simulink library "invLib"  (R2026a)
settings: Solver=VariableStepAuto
values from neighbouring files (symbols this model uses):
  ip = invParams()    [invSim.m]    (also in inv_current_loop_check.m; inv_grid_thd_check.m; inv_model_check.m; inv_thd_check.m)
libraries: nesl_utility x15, ee_lib x9, fl_lib x9, slpidlib x2
settings Model: Creator=phamn  LastModifiedBy=phamn

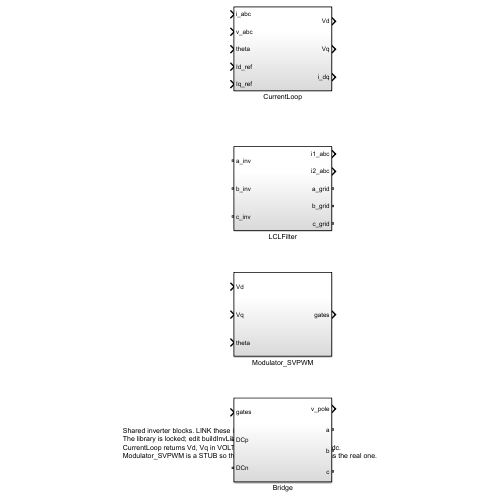
[thumbnail: Simulink's stored preview of the top-level diagram]
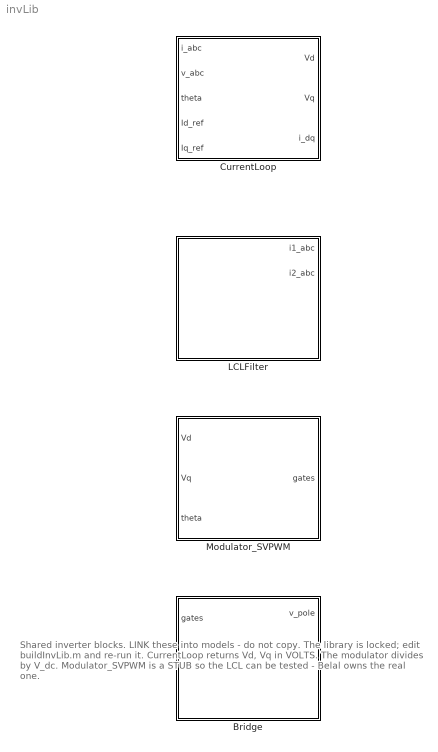
== system invLib ==
  note: Shared inverter blocks. LINK these into models - do not copy.
      | The library is locked; edit buildInvLib.m and re-run it.
      | CurrentLoop returns Vd, Vq in VOLTS. The modulator divides by V_dc.
      | Modulator_SVPWM is a STUB so the LCL can be tested - Belal owns the real one.
  Bridge : Subsystem
  CurrentLoop : Subsystem
  LCLFilter : Subsystem
  Modulator_SVPWM : Subsystem

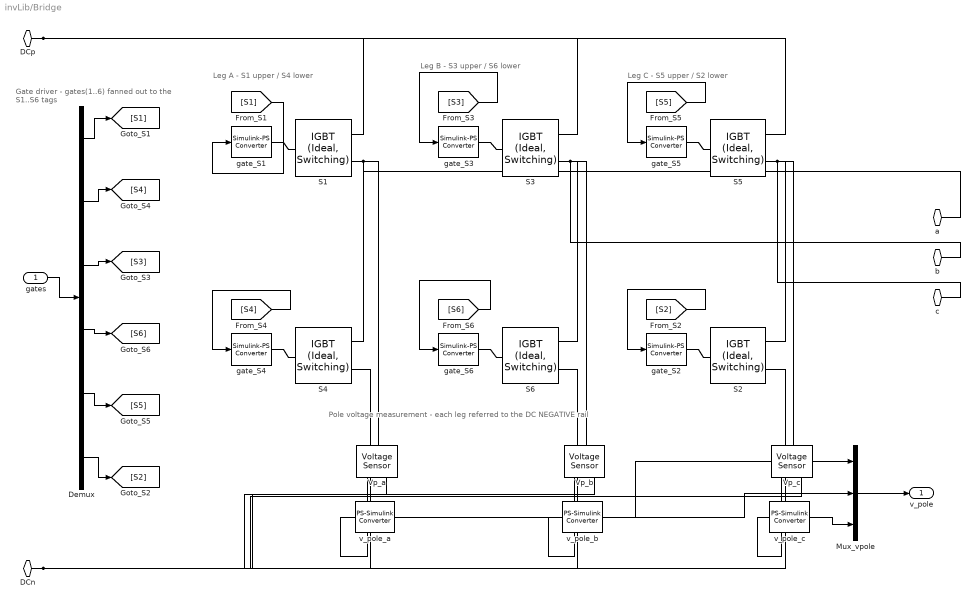
== system invLib/Bridge ==
  note: Gate driver - gates(1..6) fanned out to the S1..S6 tags
  note: Leg A - S1 upper / S4 lower
  note: Leg B - S3 upper / S6 lower
  note: Leg C - S5 upper / S2 lower
  note: Pole voltage measurement - each leg referred to the DC NEGATIVE rail
  gates : Inport
  Demux : Demux  Outputs=6
  Mux_vpole : Mux  Inputs=3
  S{1..6} (6 alike) : ee_lib/Semiconductors & Converters/IGBT (Ideal, Switching)  port_option=ee.enum.controlport.ps  Vf=ip.Vf_dev V  Ron=ip.Ron_dev Ohm  Goff=ip.Goff_dev 1/Ohm  Vth=ip.Vth_gate V  diode_param=ee.enum.semiconductors.protectionDiode.nodynamics  diode_Vf=ip.Vf_dev V  diode_Ron=ip.Ron_dev Ohm  diode_Goff=ip.Goff_dev 1/Ohm  diode_C=50e-9 F  diode_iRM=-235 A  diode_iF=300 A  diode_idot=-50 A/us  diode_trr_param=ee.enum.converters.diodeReverseParam.trr_factor  diode_trr_factor=3  diode_trr=15 us  diode_Qrr=1500 s*uA  ice_specify=off  ice_priority=None  ice=0 A  ice_nominal_specify=off  ice_nominal_value=1  ice_nominal_unit=A  vce_specify=off  vce_priority=None  vce=0 V  vce_nominal_specify=off  vce_nominal_value=1  vce_nominal_unit=V  vge_specify=off  vge_priority=None  vge=0 V  vge_nominal_specify=off  vge_nominal_value=1  vge_nominal_unit=V  thermal_loss_option=ee.enum.converters.thermalLossOption.constantvalues  Von_data=[0, .1, .6, .8, 1, 1.3, 1.6, 2, 2.4; 0, .1, .7, 1, 1.2, 1.5, 1.9, 2.4, 2.8] V  Tj=[298.15, 398.15] K  Iout_data=[0, .1, 1, 5, 10, 20, 40, 70, 100] A  tabulateWithVce=false  Eon_data=[0, .0024, .024, .12, .2, .48, 1.04, 2.16, 3.24; 0, .003, .03, .15, .25, .6, 1.3, 2.7, 4.05] * 1e-3 J  Eoff_data=[0, .0007, .0066, .033, .066, .17, .33, .83, 1.5; 0, .001, .01, .05, .1, .25, .5, 1.2, 2.2] * 1e-3 J  Eon_data_3D=[zeros(2, 9, 3)] J  Eoff_data_3D=[zeros(2, 9, 3)] J  Tj_loss=[298.15, 398.15] K  Iout_data_loss=[0, .1, 1, 5, 10, 20, 40, 70, 100] A  Vce_loss=[0, 150, 300] V  Eon_scalar=22.86e-3 J  Eoff_scalar=17.14e-3 J  Voff=300 V  Iout_scalar=600 A  useCurrentFromPreviousCycle=false  useVoltageFromPreviousCycle=false  diodeModelType=ee.enum.converters.diodeModelType.pwl  diodeTableType=ee.enum.diode.tableType.IfMat  diode_ReverseIVType=ee.enum.diode.diodeReverseIV.constant  diode_IfMat=[.07, .12, .19, 1.75, 4.24, 7.32, 11.2; .16, .3, .72, 2.14, 4.02, 6.35, 9.12] A  diode_VfMat=[.9, 1.15, 1.25, 1.5, 1.75, 2.17, 2.6, 2.85; .58, .68, .75, 1.1, 1.38, 1.77, 2.27, 2.7] V  diode_TjVec=[25, 125] degC  diode_VfVec=[.5, .7, .9, 1.3, 1.7, 2.1, 2.5] V  diode_IfVec=[.1, .2, .5, 1, 2, 4, 7, 10] A  diode_IrMat=[1e-06, 2e-06, 5e-06, 1e-05, 2.5e-05, 5e-05, .0001; 2e-06, 5e-06, 1e-05, 4e-05, 8e-05, .0002, .0005] A  diode_VrMat=[10, 100, 200, 250, 300, 325, 350; 10, 70, 160, 220, 270, 300, 320] V  diode_VrVec=[10, 20, 40, 50, 70, 80, 100] V  diode_IrVec=[1e-06, 2e-06, 5e-06, 1e-05, 2e-05, 5e-05, .0001] A  diode_Vr=-600 V  diode_Ls=150 nH  diode_Erec=0.03 J  diode_rec_loss_model=ee.enum.diode.reverseRecoveryModelTabulateUpTo3D.fixed  diode_ErecVal=0 J  diode_scaleWithIandV=true  diode_ErecMat=zeros(2, 3) J  diodeErecMat3D=zeros(2, 3, 2) J  diode_TjrecVec=[298.15, 398.15] K  diode_IfrecVec=[.1, 1, 10] A  diodeVrecVec=[0, 100] V  diode_IrecVal=10 A  diode_VrecVal=10 V  diode_tFilter=1 / 1000 / 100 s  separateThermalPortForDiode=false  thermal_network_parameterization=ee.enum.thermalNetworkTopology.external  Rth=[.08, .5] K/W  Rth_Cauer=[.08, .1, .5] K/W  Rth_Foster=[.08, .14, .22, .16] K/W  thermal_mass_parameterization=ee.enum.thermalNetwork.timeconstant  thermal_mass=[.01, .5] J/K  thermal_mass_Cauer=[.01, .1, .5] J/K  thermal_mass_Foster=[.001, .005, .05, .5] J/K  thermal_time_constant=[.001, .2] s  thermal_time_constant_Cauer=[.001, .1, .2] s  thermal_time_constant_Foster=[7e-05, .0007, .01, .08] s  thermal_mass_initial_temperatures=[25, 25] degC  thermal_mass_initial_temperatures_Cauer=[25, 25, 25] degC  junction_thermal_mass=0.01 J/K  Tvec_initial_Foster=[25, 25, 25, 25] degC  RthDiode=[.03, .2] K/W  RthCauerDiode=[.03, .1, .2] K/W  RthFosterDiode=[.03, .2] K/W  thermalMassDiode=[3, 25] J/K  thermalMassCauerDiode=[3, 10, 25] J/K  thermalMassFosterDiode=[33, 50] J/K  thermalTauDiode=[.1, 5] s  thermalTauCauerDiode=[.1, 1, 5] s  thermalTauFosterDiode=[1, 10] s  thermalMassInitTempDiode=[25, 25] degC  thermalMassInitTempCauerDiode=[25, 25, 25] degC  junctionthermalMassDiode=0.1 J/K  TVecInitialFosterDiode=[25, 25, 25, 25] degC  no_thermal_network=ee.enum.enable.no  IGBT_junction_temperature_specify=off  IGBT_junction_temperature_priority=None  IGBT_junction_temperature=25 degC  IGBT_junction_temperature_nominal_specify=off  IGBT_junction_temperature_nominal_value=1  IGBT_junction_temperature_nominal_unit=degC  diode_junction_temperature_specify=off  diode_junction_temperature_priority=None  diode_junction_temperature=25 degC  diode_junction_temperature_nominal_specify=off  diode_junction_temperature_nominal_value=1  diode_junction_temperature_nominal_unit=degC  Qj_specify=off  Qj_priority=None  Qj=0 W  Qj_nominal_specify=off  Qj_nominal_value=1  Qj_nominal_unit=W  accumulatedSwitchingLosses_specify=off  accumulatedSwitchingLosses_priority=None  accumulatedSwitchingLosses=0 J
  Vp_a : fl_lib/Electrical/Electrical Sensors/Voltage Sensor
  Vp_b : fl_lib/Electrical/Electrical Sensors/Voltage Sensor
  Vp_c : fl_lib/Electrical/Electrical Sensors/Voltage Sensor
  gate_S{1..6} (6 alike) : nesl_utility/Simulink-PS Converter  PhysicalDomain=network_engine_domain  SubClassName=ps_input  LeftPortType=input  RightPortType=output  PseudoPeriodic=off  Frequencies=[]  NoiseDistribution=none  NoiseParameters=[]  Unit=1  AffineConversion=off  FilteringAndDerivatives=provide  SimscapeFilterOrder=1  InputFilterTimeConstant=0.001  UdotUserProvided=0
  v_pole_a : nesl_utility/PS-Simulink Converter  PhysicalDomain=network_engine_domain  SubClassName=ps_output  LeftPortType=input  RightPortType=output  PseudoPeriodic=off  Frequencies=[]  VectorFormat=inherit  Unit=inherit  AffineConversion=off
  v_pole_b : nesl_utility/PS-Simulink Converter  PhysicalDomain=network_engine_domain  SubClassName=ps_output  LeftPortType=input  RightPortType=output  PseudoPeriodic=off  Frequencies=[]  VectorFormat=inherit  Unit=inherit  AffineConversion=off
  v_pole_c : nesl_utility/PS-Simulink Converter  PhysicalDomain=network_engine_domain  SubClassName=ps_output  LeftPortType=input  RightPortType=output  PseudoPeriodic=off  Frequencies=[]  VectorFormat=inherit  Unit=inherit  AffineConversion=off
  DCp : PMIOPort  Side=Left
  DCn : PMIOPort  Port=2  Side=Left
  a : PMIOPort  Port=3  Side=Right
  b : PMIOPort  Port=4  Side=Right
  c : PMIOPort  Port=5  Side=Right
  v_pole : Outport
  wires:
  gates/1 -> Demux/1
  Demux/1 -> [S1]
  Demux/2 -> [S4]
  Demux/3 -> [S3]
  Demux/4 -> [S6]
  Demux/5 -> [S5]
  Demux/6 -> [S2]
  [S1] -> gate_S1/1
  [S4] -> gate_S4/1
  v_pole_a/1 -> Mux_vpole/1
  [S3] -> gate_S3/1
  [S6] -> gate_S6/1
  v_pole_b/1 -> Mux_vpole/2
  [S5] -> gate_S5/1
  [S2] -> gate_S2/1
  v_pole_c/1 -> Mux_vpole/3
  Mux_vpole/1 -> v_pole/1
  connections:
  gate_S1/RConn1 -- S1/LConn1
  gate_S4/RConn1 -- S4/LConn1
  S1/RConn1 -- DCp/RConn1 -- S3/RConn1 -- S5/RConn1
  S4/RConn1 -- S1/RConn2 -- a/RConn1 -- Vp_a/LConn1
  S4/RConn2 -- Vp_a/RConn2 -- S6/RConn2 -- Vp_b/RConn2 -- S2/RConn2 -- DCn/RConn1 -- Vp_c/RConn2
  Vp_a/RConn1 -- v_pole_a/LConn1
  gate_S3/RConn1 -- S3/LConn1
  gate_S6/RConn1 -- S6/LConn1
  S6/RConn1 -- S3/RConn2 -- b/RConn1 -- Vp_b/LConn1
  Vp_b/RConn1 -- v_pole_b/LConn1
  gate_S5/RConn1 -- S5/LConn1
  gate_S2/RConn1 -- S2/LConn1
  S2/RConn1 -- S5/RConn2 -- c/RConn1 -- Vp_c/LConn1
  Vp_c/RConn1 -- v_pole_c/LConn1

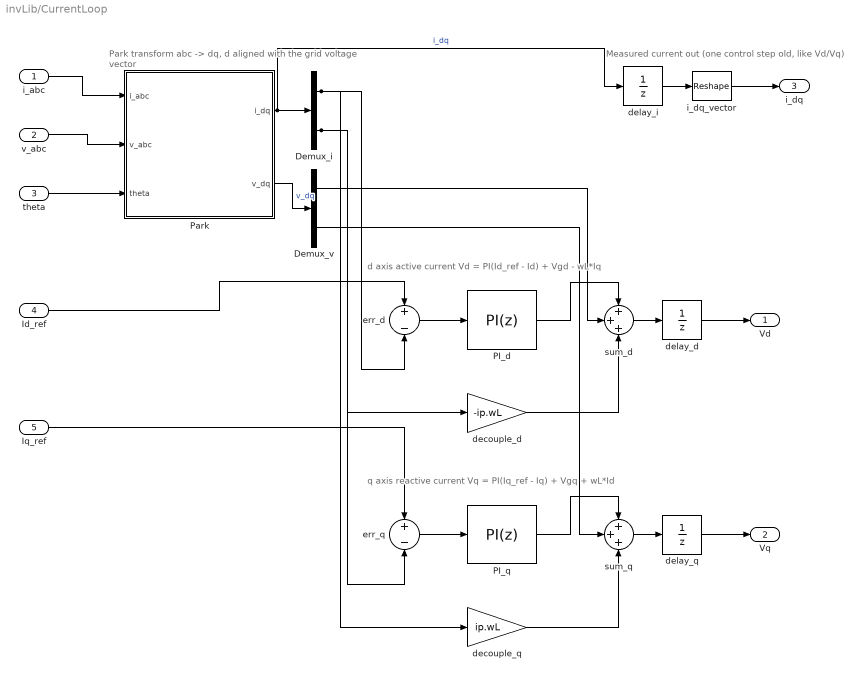
== system invLib/CurrentLoop ==
  note: Park transform abc -> dq, d aligned with the grid voltage vector
  note: d axis active current Vd = PI(Id_ref - Id) + Vgd - wL*Iq
  note: q axis reactive current Vq = PI(Iq_ref - Iq) + Vgq + wL*Id
  note: Measured current out (one control step old, like Vd/Vq)
  i_abc : Inport
  v_abc : Inport  Port=2
  theta : Inport  Port=3
  Id_ref : Inport  Port=4
  Iq_ref : Inport  Port=5
  Demux_i : Demux  Outputs=2
  Demux_v : Demux  Outputs=2
  PI_d : slpidlib/PID Controller  Controller=PI  Form=Parallel  TimeDomain=Discrete-time  UseExternalTs=off  SampleTime=ip.Ts_ctrl  IntegratorMethod=Backward Euler  FilterMethod=Forward Euler  ControllerParametersSource=internal  P=ip.Kp_i  I=ip.Ki_i  UseKiTs=off  D=0  UseExternalDerivativeSource=off  N=100  UseFilter=on  TunerSelectOption=Transfer Function Based (PID Tuner App)  InitialConditionSource=internal  InitialConditionForIntegrator=0  InitialConditionForFilter=0  DifferentiatorICPrevScaledInput=0  ExternalReset=none  TrackingMode=off  Kt=1  LimitOutput=on  SatLimitsSource=internal  UpperSaturationLimit=ip.V_pi_max  LowerSaturationLimit=-ip.V_pi_max  LinearizeAsGain=off  AntiWindupMode=clamping  Kb=1  LimitIntegrator=off  UpperIntegratorSaturationLimit=inf  LowerIntegratorSaturationLimit=-inf  POutMin=[]  POutMax=[]  IOutMin=[]  IOutMax=[]  DOutMin=[]  DOutMax=[]  NOutMin=[]  NOutMax=[]  SumOutMin=[]  SumOutMax=[]  SaturationOutMin=[]  SaturationOutMax=[]  PParamMin=[]  PParamMax=[]  IParamMin=[]  IParamMax=[]  DParamMin=[]  DParamMax=[]  NParamMin=[]  NParamMax=[]  KbParamMin=[]  KbParamMax=[]  KtParamMin=[]  KtParamMax=[]  KbOutMin=[]  KbOutMax=[]  KtOutMin=[]  KtOutMax=[]  IntegratorOutMin=[]  IntegratorOutMax=[]  FilterOutMin=[]  FilterOutMax=[]  SumI1OutMin=[]  SumI1OutMax=[]  SumI2OutMin=[]  SumI2OutMax=[]  SumI3OutMin=[]  SumI3OutMax=[]  SumI4OutMin=[]  SumI4OutMax=[]  SumDOutMin=[]  SumDOutMax=[]  DifferentiatorOutMin=[]  DifferentiatorOutMax=[]  FilterDiffOutCoefMin=[]  FilterDiffOutCoefMax=[]  ReciprocalOutMin=[]  ReciprocalOutMax=[]  SumDenOutMin=[]  SumDenOutMax=[]  SumNumOutMin=[]  SumNumOutMax=[]  DivideOutMin=[]  DivideOutMax=[]  UdiffTsProdOutMin=[]  UdiffTsProdOutMax=[]  NTsProdOutMin=[]  NTsProdOutMax=[]  UintegralTsProdOutMin=[]  UintegralTsProdOutMax=[]  UngainTsProdOutMin=[]  UngainTsProdOutMax=[]  ClampingZeroOutDataTypeStr=Inherit: Inherit via back propagation  ClampingZeroOutMin=[]  ClampingZeroOutMax=[]  FilterDenConstantOutDataTypeStr=Inherit: Inherit via back propagation  FilterDenConstantOutMin=[]  FilterDenConstantOutMax=[]  PCopyOutDataTypeStr=Inherit: Inherit via back propagation  PCopyOutMin=[]  PCopyOutMax=[]  NCopyOutDataTypeStr=Inherit: Inherit via back propagation  NCopyOutMin=[]  NCopyOutMax=[]  IntegratorContinuousStateAttributes=''  IntegratorStateMustResolveToSignalObject=off  IntegratorRTWStateStorageClass=Auto  FilterContinuousStateAttributes=''  FilterStateMustResolveToSignalObject=off  FilterRTWStateStorageClass=Auto  ParallelPVariant=InternalParameters  IdealPVariant=Disabled  IVariant=InternalParameters  DVariant=Disabled  IntegratorVariant=Discrete  SatVariant=Enabled  AWVariant=DiscClampingParallel  PCopyVariant=Disabled  TRVariant=Disabled  FdbkBlocksVariant=Feedback  IdealPFdbkVariant=Passthrough  SatFdbkVariant=Passthrough  DerivativeFilterVariant=Disabled  NVariant=Disabled  NCopyVariant=Disabled_SignalSpec  FilterICVariant=Disabled  IntegratorICVariant=InternalICs  ExternalResetVariant=Disabled  TRSumVariant=Passthrough  SumFdbkVariant=Enabled  SumVariant=Sum_PI  TsampFilterVariant=InternalTs  TsampNgainVariant=Passthrough  TsampIntegralVariant=Disabled_SignalSpec  ExternalSaturationOutDataTypeStr=Inherit: Same as second input  DerivativeSourceVariant=Disabled  PreIntVariant=InternalPreInt
      settings: LibrarySourceBlock=simulink/Discrete/Discrete PID Controller
  PI_q : slpidlib/PID Controller  Controller=PI  Form=Parallel  TimeDomain=Discrete-time  UseExternalTs=off  SampleTime=ip.Ts_ctrl  IntegratorMethod=Backward Euler  FilterMethod=Forward Euler  ControllerParametersSource=internal  P=ip.Kp_i  I=ip.Ki_i  UseKiTs=off  D=0  UseExternalDerivativeSource=off  N=100  UseFilter=on  TunerSelectOption=Transfer Function Based (PID Tuner App)  InitialConditionSource=internal  InitialConditionForIntegrator=0  InitialConditionForFilter=0  DifferentiatorICPrevScaledInput=0  ExternalReset=none  TrackingMode=off  Kt=1  LimitOutput=on  SatLimitsSource=internal  UpperSaturationLimit=ip.V_pi_max  LowerSaturationLimit=-ip.V_pi_max  LinearizeAsGain=off  AntiWindupMode=clamping  Kb=1  LimitIntegrator=off  UpperIntegratorSaturationLimit=inf  LowerIntegratorSaturationLimit=-inf  POutMin=[]  POutMax=[]  IOutMin=[]  IOutMax=[]  DOutMin=[]  DOutMax=[]  NOutMin=[]  NOutMax=[]  SumOutMin=[]  SumOutMax=[]  SaturationOutMin=[]  SaturationOutMax=[]  PParamMin=[]  PParamMax=[]  IParamMin=[]  IParamMax=[]  DParamMin=[]  DParamMax=[]  NParamMin=[]  NParamMax=[]  KbParamMin=[]  KbParamMax=[]  KtParamMin=[]  KtParamMax=[]  KbOutMin=[]  KbOutMax=[]  KtOutMin=[]  KtOutMax=[]  IntegratorOutMin=[]  IntegratorOutMax=[]  FilterOutMin=[]  FilterOutMax=[]  SumI1OutMin=[]  SumI1OutMax=[]  SumI2OutMin=[]  SumI2OutMax=[]  SumI3OutMin=[]  SumI3OutMax=[]  SumI4OutMin=[]  SumI4OutMax=[]  SumDOutMin=[]  SumDOutMax=[]  DifferentiatorOutMin=[]  DifferentiatorOutMax=[]  FilterDiffOutCoefMin=[]  FilterDiffOutCoefMax=[]  ReciprocalOutMin=[]  ReciprocalOutMax=[]  SumDenOutMin=[]  SumDenOutMax=[]  SumNumOutMin=[]  SumNumOutMax=[]  DivideOutMin=[]  DivideOutMax=[]  UdiffTsProdOutMin=[]  UdiffTsProdOutMax=[]  NTsProdOutMin=[]  NTsProdOutMax=[]  UintegralTsProdOutMin=[]  UintegralTsProdOutMax=[]  UngainTsProdOutMin=[]  UngainTsProdOutMax=[]  ClampingZeroOutDataTypeStr=Inherit: Inherit via back propagation  ClampingZeroOutMin=[]  ClampingZeroOutMax=[]  FilterDenConstantOutDataTypeStr=Inherit: Inherit via back propagation  FilterDenConstantOutMin=[]  FilterDenConstantOutMax=[]  PCopyOutDataTypeStr=Inherit: Inherit via back propagation  PCopyOutMin=[]  PCopyOutMax=[]  NCopyOutDataTypeStr=Inherit: Inherit via back propagation  NCopyOutMin=[]  NCopyOutMax=[]  IntegratorContinuousStateAttributes=''  IntegratorStateMustResolveToSignalObject=off  IntegratorRTWStateStorageClass=Auto  FilterContinuousStateAttributes=''  FilterStateMustResolveToSignalObject=off  FilterRTWStateStorageClass=Auto  ParallelPVariant=InternalParameters  IdealPVariant=Disabled  IVariant=InternalParameters  DVariant=Disabled  IntegratorVariant=Discrete  SatVariant=Enabled  AWVariant=DiscClampingParallel  PCopyVariant=Disabled  TRVariant=Disabled  FdbkBlocksVariant=Feedback  IdealPFdbkVariant=Passthrough  SatFdbkVariant=Passthrough  DerivativeFilterVariant=Disabled  NVariant=Disabled  NCopyVariant=Disabled_SignalSpec  FilterICVariant=Disabled  IntegratorICVariant=InternalICs  ExternalResetVariant=Disabled  TRSumVariant=Passthrough  SumFdbkVariant=Enabled  SumVariant=Sum_PI  TsampFilterVariant=InternalTs  TsampNgainVariant=Passthrough  TsampIntegralVariant=Disabled_SignalSpec  ExternalSaturationOutDataTypeStr=Inherit: Same as second input  DerivativeSourceVariant=Disabled  PreIntVariant=InternalPreInt
      settings: LibrarySourceBlock=simulink/Discrete/Discrete PID Controller
  Park : MATLAB Function  TreatAsAtomicUnit=on
  decouple_d : Gain  Gain=-ip.wL
  decouple_q : Gain  Gain=ip.wL
  delay_d : UnitDelay  SampleTime=ip.Ts_ctrl
  delay_i : UnitDelay  SampleTime=ip.Ts_ctrl
  delay_q : UnitDelay  SampleTime=ip.Ts_ctrl
  err_d : Sum  Inputs=+-
  err_q : Sum  Inputs=+-
  i_dq_vector : Reshape
  sum_d : Sum  Inputs=+++
  sum_q : Sum  Inputs=+++
  Vd : Outport
  Vq : Outport  Port=2
  i_dq : Outport  Port=3
  wires:
  i_abc/1 -> Park/1(i_abc)
  v_abc/1 -> Park/2(v_abc)
  theta/1 -> Park/3(theta)
  Park/1(i_dq) -> Demux_i/1, delay_i/1  "i_dq"
  Park/2(v_dq) -> Demux_v/1  "v_dq"
  Id_ref/1 -> err_d/1
  Demux_i/1 -> err_d/2, decouple_q/1
  Iq_ref/1 -> err_q/1
  Demux_i/2 -> err_q/2, decouple_d/1
  err_d/1 -> PI_d/1
  err_q/1 -> PI_q/1
  PI_d/1 -> sum_d/1
  Demux_v/1 -> sum_d/2
  decouple_d/1 -> sum_d/3
  PI_q/1 -> sum_q/1
  Demux_v/2 -> sum_q/2
  decouple_q/1 -> sum_q/3
  sum_d/1 -> delay_d/1
  sum_q/1 -> delay_q/1
  delay_d/1 -> Vd/1
  delay_q/1 -> Vq/1
  delay_i/1 -> i_dq_vector/1
  i_dq_vector/1 -> i_dq/1

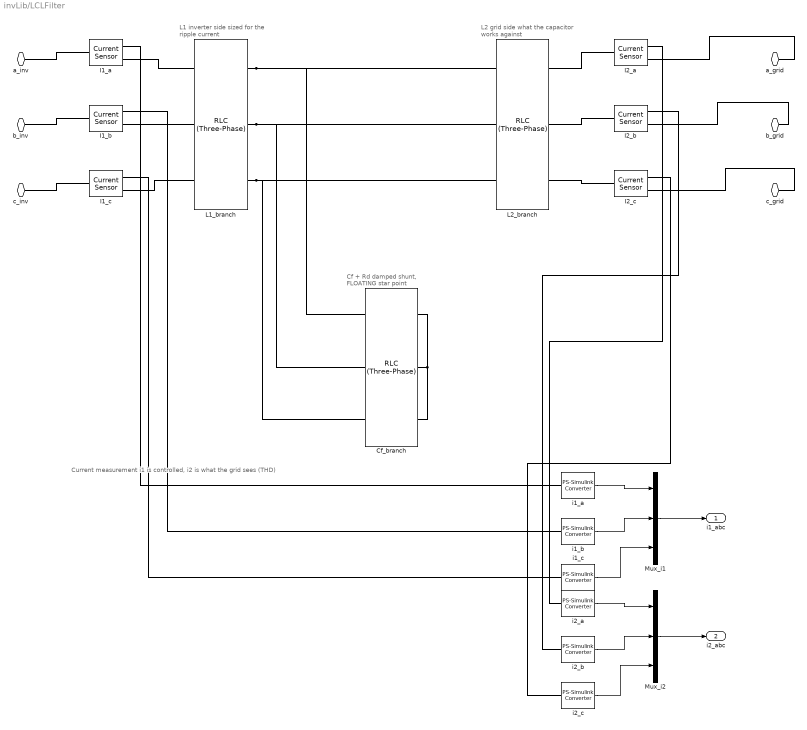
== system invLib/LCLFilter ==
  note: L1 inverter side sized for the ripple current
  note: Cf + Rd damped shunt, FLOATING star point
  note: L2 grid side what the capacitor works against
  note: Current measurement i1 is controlled, i2 is what the grid sees (THD)
  Cf_branch : ee_lib/Passive/RLC Assemblies/RLC (Three-Phase)  port_option=ee.enum.threePhasePort.expanded  component_structure=ee.enum.rlc.structure.SeriesRC  R=ip.Rd Ohm  L=ip.L1 H  C=ip.Cf F  R_parasitic=0 Ohm  G_parasitic=0 1/Ohm  IL_specify=off  IL_priority=High  IL=[0, 0, 0] A  IL_nominal_specify=off  IL_nominal_value=1  IL_nominal_unit=A  VC_specify=off  VC_priority=High  VC=[0, 0, 0] V  VC_nominal_specify=off  VC_nominal_value=1  VC_nominal_unit=V
  I1_a : fl_lib/Electrical/Electrical Sensors/Current Sensor
  I1_b : fl_lib/Electrical/Electrical Sensors/Current Sensor
  I1_c : fl_lib/Electrical/Electrical Sensors/Current Sensor
  I2_a : fl_lib/Electrical/Electrical Sensors/Current Sensor
  I2_b : fl_lib/Electrical/Electrical Sensors/Current Sensor
  I2_c : fl_lib/Electrical/Electrical Sensors/Current Sensor
  L1_branch : ee_lib/Passive/RLC Assemblies/RLC (Three-Phase)  port_option=ee.enum.threePhasePort.expanded  component_structure=ee.enum.rlc.structure.SeriesRL  R=ip.R1 Ohm  L=ip.L1 H  C=ip.Cf F  R_parasitic=0 Ohm  G_parasitic=0 1/Ohm  IL_specify=off  IL_priority=High  IL=[0, 0, 0] A  IL_nominal_specify=off  IL_nominal_value=1  IL_nominal_unit=A  VC_specify=off  VC_priority=High  VC=[0, 0, 0] V  VC_nominal_specify=off  VC_nominal_value=1  VC_nominal_unit=V
  L2_branch : ee_lib/Passive/RLC Assemblies/RLC (Three-Phase)  port_option=ee.enum.threePhasePort.expanded  component_structure=ee.enum.rlc.structure.SeriesRL  R=ip.R2 Ohm  L=ip.L2 H  C=ip.Cf F  R_parasitic=0 Ohm  G_parasitic=0 1/Ohm  IL_specify=off  IL_priority=High  IL=[0, 0, 0] A  IL_nominal_specify=off  IL_nominal_value=1  IL_nominal_unit=A  VC_specify=off  VC_priority=High  VC=[0, 0, 0] V  VC_nominal_specify=off  VC_nominal_value=1  VC_nominal_unit=V
  Mux_i1 : Mux  Inputs=3
  Mux_i2 : Mux  Inputs=3
  i1_a : nesl_utility/PS-Simulink Converter  PhysicalDomain=network_engine_domain  SubClassName=ps_output  LeftPortType=input  RightPortType=output  PseudoPeriodic=off  Frequencies=[]  VectorFormat=inherit  Unit=inherit  AffineConversion=off
  i1_b : nesl_utility/PS-Simulink Converter  PhysicalDomain=network_engine_domain  SubClassName=ps_output  LeftPortType=input  RightPortType=output  PseudoPeriodic=off  Frequencies=[]  VectorFormat=inherit  Unit=inherit  AffineConversion=off
  i1_c : nesl_utility/PS-Simulink Converter  PhysicalDomain=network_engine_domain  SubClassName=ps_output  LeftPortType=input  RightPortType=output  PseudoPeriodic=off  Frequencies=[]  VectorFormat=inherit  Unit=inherit  AffineConversion=off
  i2_a : nesl_utility/PS-Simulink Converter  PhysicalDomain=network_engine_domain  SubClassName=ps_output  LeftPortType=input  RightPortType=output  PseudoPeriodic=off  Frequencies=[]  VectorFormat=inherit  Unit=inherit  AffineConversion=off
  i2_b : nesl_utility/PS-Simulink Converter  PhysicalDomain=network_engine_domain  SubClassName=ps_output  LeftPortType=input  RightPortType=output  PseudoPeriodic=off  Frequencies=[]  VectorFormat=inherit  Unit=inherit  AffineConversion=off
  i2_c : nesl_utility/PS-Simulink Converter  PhysicalDomain=network_engine_domain  SubClassName=ps_output  LeftPortType=input  RightPortType=output  PseudoPeriodic=off  Frequencies=[]  VectorFormat=inherit  Unit=inherit  AffineConversion=off
  a_inv : PMIOPort  Side=Left
  b_inv : PMIOPort  Port=2  Side=Left
  c_inv : PMIOPort  Port=3  Side=Left
  a_grid : PMIOPort  Port=4  Side=Right
  b_grid : PMIOPort  Port=5  Side=Right
  c_grid : PMIOPort  Port=6  Side=Right
  i1_abc : Outport
  i2_abc : Outport  Port=2
  wires:
  i1_a/1 -> Mux_i1/1
  i2_a/1 -> Mux_i2/1
  i1_b/1 -> Mux_i1/2
  i2_b/1 -> Mux_i2/2
  i1_c/1 -> Mux_i1/3
  i2_c/1 -> Mux_i2/3
  Mux_i1/1 -> i1_abc/1
  Mux_i2/1 -> i2_abc/1
  connections:
  a_inv/RConn1 -- I1_a/LConn1
  I1_a/RConn2 -- L1_branch/LConn1
  Cf_branch/LConn1 -- L1_branch/RConn1 -- L2_branch/LConn1
  L2_branch/RConn1 -- I2_a/LConn1
  I2_a/RConn2 -- a_grid/RConn1
  I1_a/RConn1 -- i1_a/LConn1
  I2_a/RConn1 -- i2_a/LConn1
  b_inv/RConn1 -- I1_b/LConn1
  I1_b/RConn2 -- L1_branch/LConn2
  Cf_branch/LConn2 -- L1_branch/RConn2 -- L2_branch/LConn2
  L2_branch/RConn2 -- I2_b/LConn1
  I2_b/RConn2 -- b_grid/RConn1
  I1_b/RConn1 -- i1_b/LConn1
  I2_b/RConn1 -- i2_b/LConn1
  c_inv/RConn1 -- I1_c/LConn1
  I1_c/RConn2 -- L1_branch/LConn3
  Cf_branch/LConn3 -- L1_branch/RConn3 -- L2_branch/LConn3
  L2_branch/RConn3 -- I2_c/LConn1
  I2_c/RConn2 -- c_grid/RConn1
  I1_c/RConn1 -- i1_c/LConn1
  I2_c/RConn1 -- i2_c/LConn1
  Cf_branch/RConn2 -- Cf_branch/RConn1 -- Cf_branch/RConn3

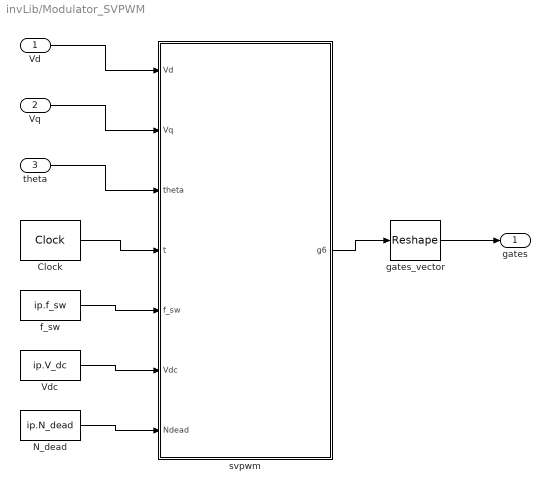
== system invLib/Modulator_SVPWM ==
  Vd : Inport
  Vq : Inport  Port=2
  theta : Inport  Port=3
  Clock : DigitalClock  SampleTime=ip.Ts_power
  N_dead : Constant  Value=ip.N_dead
  Vdc : Constant  Value=ip.V_dc
  f_sw : Constant  Value=ip.f_sw
  gates_vector : Reshape
  svpwm : MATLAB Function  TreatAsAtomicUnit=on
  gates : Outport
  wires:
  Vd/1 -> svpwm/1(Vd)
  Vq/1 -> svpwm/2(Vq)
  theta/1 -> svpwm/3(theta)
  Clock/1 -> svpwm/4(t)
  f_sw/1 -> svpwm/5(f_sw)
  Vdc/1 -> svpwm/6(Vdc)
  N_dead/1 -> svpwm/7(Ndead)
  svpwm/1(g6) -> gates_vector/1
  gates_vector/1 -> gates/1

== matlab function invLib/Modulator_SVPWM/svpwm ==
  data: Vd input; g6 output; Vq input; theta input; t input; f_sw input; Vdc input; Ndead input
function g6 = svpwm(Vd, Vq, theta, t, f_sw, Vdc, Ndead)
%#codegen
% SVPWM by min-max zero-sequence injection, with dead time.
%
% STUB - Belal owns the real modulator. This is a correct SVPWM rather than a
% placeholder: min-max injection is mathematically identical to classical
% sector-and-timing SVPWM and reaches the same V_dc/sqrt(3) ceiling.
persistent gprev cnt
if isempty(gprev)
    gprev = zeros(3,1);
    cnt   = Ndead*ones(3,1);        % start with the blanking already expired
end

v = [ Vd*cos(theta)         - Vq*sin(theta); ...
      Vd*cos(theta-2*pi/3)  - Vq*sin(theta-2*pi/3); ...
      Vd*cos(theta+2*pi/3)  - Vq*sin(theta+2*pi/3) ];

% Zero-sequence injection. Common to all three phases, so it cancels in every
% line-to-line voltage and drives no current in a three-wire system - it only
% buys headroom, and that headroom IS the 15.5%% SVPWM has over SPWM.
v = v - (max(v) + min(v))/2;

m = v/(Vdc/2);                      % per-leg modulation index
m = min(max(m, -1), 1);             % clip; overmodulation is not modelled

frac = t*f_sw - floor(t*f_sw);      % triangular carrier, -1 .. 1
tri  = 4*abs(frac - 0.5) - 1;
g    = double(m > tri);             % raw leg command, 1 = upper on

% Dead time: on any leg transition blank BOTH devices for Ndead steps.
g6 = zeros(6,1);
for k = 1:3
    if g(k) ~= gprev(k)
        cnt(k) = 0;
    elseif cnt(k) < Ndead
        cnt(k) = cnt(k) + 1;
    end
    live = cnt(k) >= Ndead;
    g6(2*k-1) = double(g(k) == 1 && live);      % upper
    g6(2*k)   = double(g(k) == 0 && live);      % lower
end
gprev = g;

== matlab function invLib/CurrentLoop/Park ==
  data: i_abc input; i_dq output; v_abc input; theta input; v_dq output
function [i_dq, v_dq] = park(i_abc, v_abc, theta)
%#codegen
% Amplitude-invariant Park transform, d aligned with the grid voltage vector.
%
% With theta the grid angle from the PLL, a balanced grid gives v_dq = [Vpk; 0],
% so Id is the active current and Iq the reactive current. Amplitude-invariant
% (the 2/3 scaling) means Id is a real amperes peak, not a scaled quantity -
% the current limit and the rating are then the same number everywhere.
c = [cos(theta), cos(theta - 2*pi/3), cos(theta + 2*pi/3)];
s = [sin(theta), sin(theta - 2*pi/3), sin(theta + 2*pi/3)];
i_dq = (2/3)*[ c*i_abc(:); -s*i_abc(:) ];
v_dq = (2/3)*[ c*v_abc(:); -s*v_abc(:) ];
